simulink model "tutorial23_mrac"  (R2025a)
settings: Solver=VariableStepAuto  StartTime=0.0  StopTime=10.0  RelTol=1e-3
settings Model: Creator=xing2  LastModifiedBy=xing2

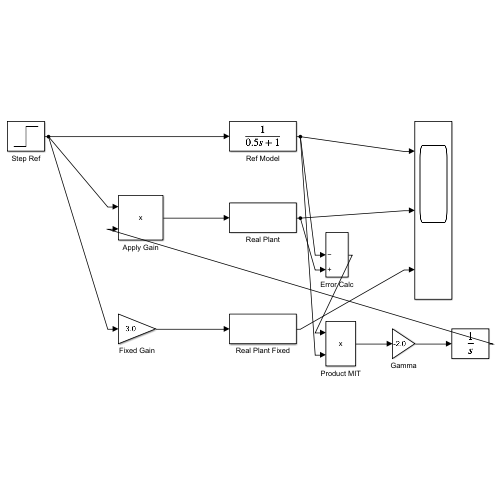
[thumbnail: Simulink's stored preview of the top-level diagram]
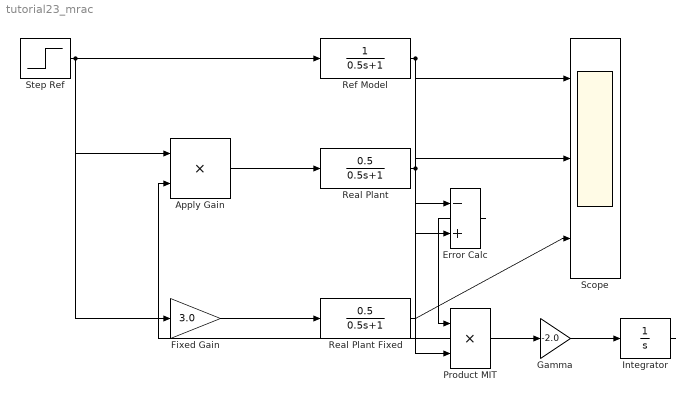
== system tutorial23_mrac ==
  Apply Gain : Product
  Error Calc : Sum  Inputs=|-+
  Fixed Gain : Gain  Gain=3.0
  Gamma : Gain  Gain=-2.0
  Integrator : Integrator  InitialCondition=1.0
  Product MIT : Product
  Real Plant : TransferFcn  Numerator=0.5  Denominator=[0.5 1]
  Real Plant Fixed : TransferFcn  Numerator=0.5  Denominator=[0.5 1]
  Ref Model : TransferFcn  Numerator=1  Denominator=[0.5 1]
  Scope : Scope  NumInputPorts=3
  Step Ref : Step  Time=0.5  After=2  SampleTime=0
  wires:
  Step Ref/1 -> Ref Model/1, Apply Gain/1, Fixed Gain/1
  Ref Model/1 -> Scope/1, Error Calc/1, Product MIT/2
  Apply Gain/1 -> Real Plant/1
  Real Plant/1 -> Scope/2, Error Calc/2
  Fixed Gain/1 -> Real Plant Fixed/1
  Real Plant Fixed/1 -> Scope/3
  Error Calc/1 -> Product MIT/1
  Product MIT/1 -> Gamma/1
  Gamma/1 -> Integrator/1
  Integrator/1 -> Apply Gain/2
